simulink model "Controllers"  (R2020b)
settings: Solver=VariableStepAuto  StartTime=0.0  StopTime=10.0  RelTol=1e-3
model workspace (MAT data in the model file):
  MPlanned = Simulink.Parameter
  MPlanned.Value = 0
  MPlanned.DataType = 'auto'
  MPlanned.Dimensions = [1 1]
undefined symbols (not defined in the file): dt
libraries: RRProbotLibrary x3
settings Model: DataDictionary=RRProbotDictionary.sldd  EnableAccessToBaseWorkspace=off  ParameterArgumentNames=MPlanned  OrderedModelArguments=off  Creator=alons  LastModifiedBy=alons

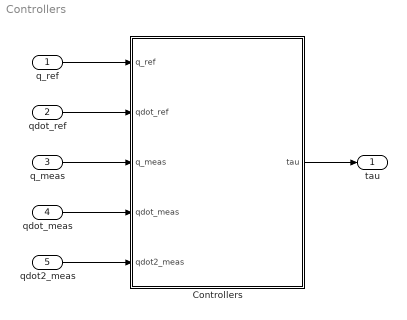
== system Controllers ==
  q_ref : Inport  PortDimensions=3
  qdot_ref : Inport  Port=2  PortDimensions=3
  q_meas : Inport  Port=3  PortDimensions=3
  qdot_meas : Inport  Port=4  PortDimensions=3
  qdot2_meas : Inport  Port=5  PortDimensions=3
  Controllers : Subsystem  Variant=on  VariantControlMode=label  VariantControl=Choice  LabelModeActiveChoice=Choice
  tau : Outport  PortDimensions=3
  wires:
  q_ref/1 -> Controllers/1(q_ref)
  qdot_ref/1 -> Controllers/2(qdot_ref)
  q_meas/1 -> Controllers/3(q_meas)
  qdot_meas/1 -> Controllers/4(qdot_meas)
  qdot2_meas/1 -> Controllers/5(qdot2_meas)
  Controllers/1(tau) -> tau/1

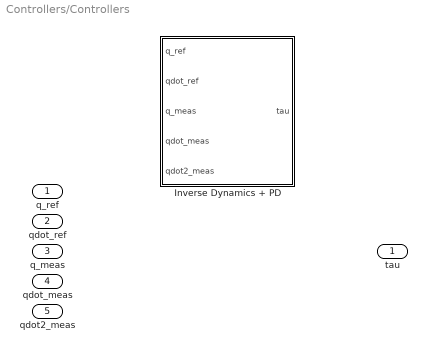
== system Controllers/Controllers ==
  q_ref : Inport
  qdot_ref : Inport  Port=2
  q_meas : Inport  Port=3
  qdot_meas : Inport  Port=4
  qdot2_meas : Inport  Port=5
  Inverse Dynamics + PD : Subsystem  VariantControl=Choice  mask{Kp=0, Kd=0, MPlanned=1}
  tau : Outport

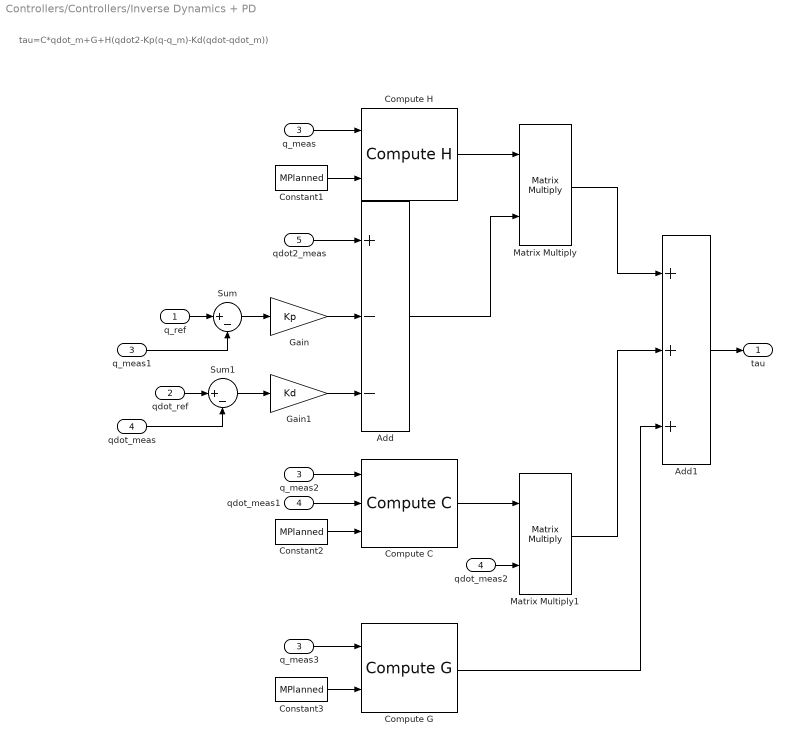
== system Controllers/Controllers/Inverse Dynamics + PD ==
  note: tau=C*qdot_m+G+H(qdot2-Kp(q-q_m)-Kd(qdot-qdot_m))
  q_ref : Inport  PortDimensions=3
  qdot_ref : Inport  Port=2  PortDimensions=3
  q_meas : Inport  Port=3  PortDimensions=3
  qdot_meas : Inport  Port=4  PortDimensions=3
  qdot2_meas : Inport  Port=5  PortDimensions=3
  Add : Sum  Inputs=+--
  Add1 : Sum  Inputs=3
  Compute C : RRProbotLibrary/Compute C  SystemSampleTime=-1  VariantActivationTime=update diagram  Latency=0  AutoFrameSizeCalculation=off
  Compute G : RRProbotLibrary/Compute G  SystemSampleTime=-1  VariantActivationTime=update diagram  Latency=0  AutoFrameSizeCalculation=off
  Compute H : RRProbotLibrary/Compute H  SystemSampleTime=-1  VariantActivationTime=update diagram  Latency=0  AutoFrameSizeCalculation=off
  Constant1 : Constant  Value=MPlanned  SampleTime=dt
  Constant2 : Constant  Value=MPlanned  SampleTime=dt
  Constant3 : Constant  Value=MPlanned  SampleTime=dt
  Gain : Gain  Gain=Kp
  Gain1 : Gain  Gain=Kd
  Matrix Multiply : Product  Multiplication=Matrix(*)
  Matrix Multiply1 : Product  Multiplication=Matrix(*)
  Sum : Sum  Inputs=|+-
  Sum1 : Sum  Inputs=|+-
  q_meas1 : InportShadow  Port=3  PortDimensions=3
  q_meas2 : InportShadow  Port=3  PortDimensions=3
  q_meas3 : InportShadow  Port=3  PortDimensions=3
  qdot_meas1 : InportShadow  Port=4  PortDimensions=3
  qdot_meas2 : InportShadow  Port=4  PortDimensions=3
  tau : Outport
  wires:
  Compute C/1 -> Matrix Multiply1/1
  q_meas/1 -> Compute H/1
  Constant1/1 -> Compute H/2
  Compute H/1 -> Matrix Multiply/1
  qdot2_meas/1 -> Add/1
  q_ref/1 -> Sum/1
  q_meas1/1 -> Sum/2
  Sum/1 -> Gain/1
  qdot_ref/1 -> Sum1/1
  qdot_meas/1 -> Sum1/2
  Sum1/1 -> Gain1/1
  Add/1 -> Matrix Multiply/2
  Constant2/1 -> Compute C/3
  qdot_meas1/1 -> Compute C/2
  q_meas2/1 -> Compute C/1
  qdot_meas2/1 -> Matrix Multiply1/2
  Gain/1 -> Add/2
  Gain1/1 -> Add/3
  q_meas3/1 -> Compute G/1
  Constant3/1 -> Compute G/2
  Matrix Multiply/1 -> Add1/1
  Matrix Multiply1/1 -> Add1/2
  Compute G/1 -> Add1/3
  Add1/1 -> tau/1
